simulink model "ClosedLoop"  (R2018b)
settings: Solver=VariableStepAuto  StartTime=0.0  StopTime=10  RelTol=1e-3
libraries: neural x533
(part 6 of 24)

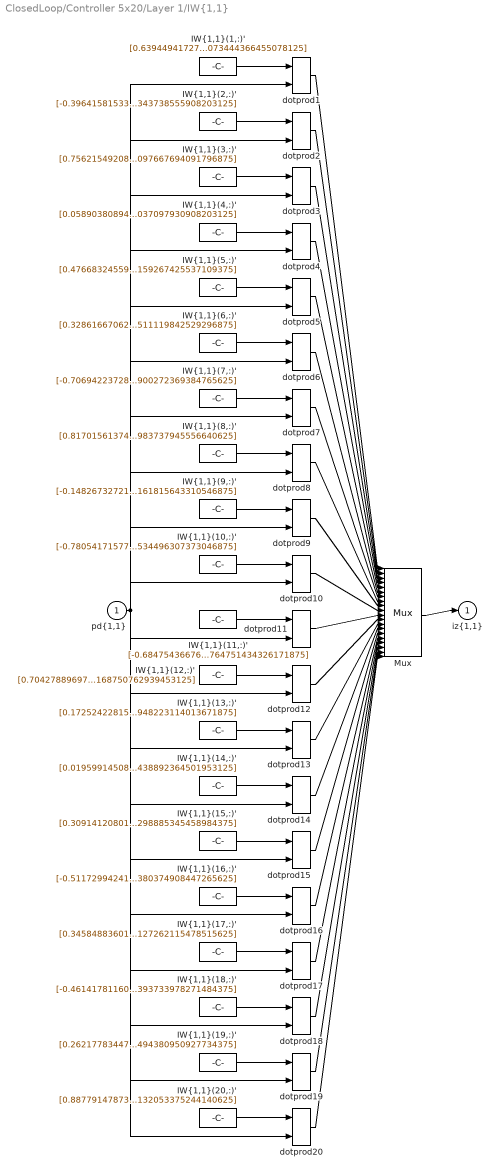
== system ClosedLoop/Controller 5x20/Layer 1/IW{1,1} ==
  "pd{1,1}" : Inport  PortDimensions=5
      mask Display: e = 0.06;c1 = [120 230 180]/255;c2 = ([120 230 180]+0)/(256+128);c3 = ([120 230 180]+128)/(256+128);patch([0 1 1 0],[0 0 1 1],c1);patch([0 1 1 1-e 1-e 0+e],[0 0 1 1-e 0+e 0+e],c2);patch([0 0 1 1-e 0+e 0+e],[0 1 1 1-e 1-e 0+e],c3);plot([0 1 1 0 0],[0 0 1 1 0]);
  "IW{1,1}(1,:)'" : Constant  Value=[0.63944941727794779584570505903684534132480621337890625;0.441873982701390388694306921024690382182598114013671875;0.1810593625517409321901141083799302577972412109375;-0.288327270168069638156538303519482724368572235107421875;-0.427441282480707507307471360036288388073444366455078125]
      mask Display: e = 0.06;c1 = [120 150 230]/255;c2 = ([120 150 230]+0)/383;c3 = ([120 150 230]+128)/383;patch([0 1 1 0],[0 0 1 1],c1);patch([0 1 1 1-e 1-e 0+e],[0 0 1 1-e 0+e 0+e],c2);patch([0 0 1 1-e 0+e 0+e],[0 1 1 1-e 1-e 0+e],c3);plot([0 1 1 0 0],[0 0 1 1 0]);disp('Weights');
  "IW{1,1}(10,:)'" : Constant  Value=[-0.780541715777256950303808480384759604930877685546875;0.64768264751365112186221040246891789138317108154296875;0.0832744460106624728723545558750629425048828125;0.52460666987157733576196960711968131363391876220703125;0.01510391606472875729305638259347688290290534496307373046875]
      mask Display: e = 0.06;c1 = [120 150 230]/255;c2 = ([120 150 230]+0)/383;c3 = ([120 150 230]+128)/383;patch([0 1 1 0],[0 0 1 1],c1);patch([0 1 1 1-e 1-e 0+e],[0 0 1 1-e 0+e 0+e],c2);patch([0 0 1 1-e 0+e 0+e],[0 1 1 1-e 1-e 0+e],c3);plot([0 1 1 0 0],[0 0 1 1 0]);disp('Weights');
  "IW{1,1}(11,:)'" : Constant  Value=[-0.68475436676158640825207157831755466759204864501953125;-0.357319180860754148643110283956048078835010528564453125;-0.6134220048648766354659755961620248854160308837890625;-0.55516072875852484624914495725533924996852874755859375;-0.47606734988326493418497875609318725764751434326171875]
      mask Display: e = 0.06;c1 = [120 150 230]/255;c2 = ([120 150 230]+0)/383;c3 = ([120 150 230]+128)/383;patch([0 1 1 0],[0 0 1 1],c1);patch([0 1 1 1-e 1-e 0+e],[0 0 1 1-e 0+e 0+e],c2);patch([0 0 1 1-e 0+e 0+e],[0 1 1 1-e 1-e 0+e],c3);plot([0 1 1 0 0],[0 0 1 1 0]);disp('Weights');
  "IW{1,1}(12,:)'" : Constant  Value=[0.70427889697472767505104229712742380797863006591796875;0.30288422449172036632347726481384597718715667724609375;-0.0523751521182032886425616879932931624352931976318359375;0.6147646637613533027177936673979274928569793701171875;0.41756010873698035101853065498289652168750762939453125]
      mask Display: e = 0.06;c1 = [120 150 230]/255;c2 = ([120 150 230]+0)/383;c3 = ([120 150 230]+128)/383;patch([0 1 1 0],[0 0 1 1],c1);patch([0 1 1 1-e 1-e 0+e],[0 0 1 1-e 0+e 0+e],c2);patch([0 0 1 1-e 0+e 0+e],[0 1 1 1-e 1-e 0+e],c3);plot([0 1 1 0 0],[0 0 1 1 0]);disp('Weights');
  "IW{1,1}(13,:)'" : Constant  Value=[0.172524228158408454714134450114215724170207977294921875;0.01229162079763308247637443315625205286778509616851806640625;-0.73979290215458792800973242265172302722930908203125;0.249500982539548832317422011328744702041149139404296875;-0.57950215730051979345915924568544141948223114013671875]
      mask Display: e = 0.06;c1 = [120 150 230]/255;c2 = ([120 150 230]+0)/383;c3 = ([120 150 230]+128)/383;patch([0 1 1 0],[0 0 1 1],c1);patch([0 1 1 1-e 1-e 0+e],[0 0 1 1-e 0+e 0+e],c2);patch([0 0 1 1-e 0+e 0+e],[0 1 1 1-e 1-e 0+e],c3);plot([0 1 1 0 0],[0 0 1 1 0]);disp('Weights');
  "IW{1,1}(14,:)'" : Constant  Value=[0.01959914508530875842939877884418820030987262725830078125;-0.682683523295935845709436762263067066669464111328125;-0.254846757327596928899282602287712506949901580810546875;-0.470498201017735373508088514427072368562221527099609375;-0.402036750942489196081197633247938938438892364501953125]
      mask Display: e = 0.06;c1 = [120 150 230]/255;c2 = ([120 150 230]+0)/383;c3 = ([120 150 230]+128)/383;patch([0 1 1 0],[0 0 1 1],c1);patch([0 1 1 1-e 1-e 0+e],[0 0 1 1-e 0+e 0+e],c2);patch([0 0 1 1-e 0+e 0+e],[0 1 1 1-e 1-e 0+e],c3);plot([0 1 1 0 0],[0 0 1 1 0]);disp('Weights');
  "IW{1,1}(15,:)'" : Constant  Value=[0.30914120801182909392679221127764321863651275634765625;-0.3889526490302082084582480092649348080158233642578125;-0.630260952151780795560398473753593862056732177734375;0.50292774374151016925083013120456598699092864990234375;0.60317210715845648305588611037819646298885345458984375]
      mask Display: e = 0.06;c1 = [120 150 230]/255;c2 = ([120 150 230]+0)/383;c3 = ([120 150 230]+128)/383;patch([0 1 1 0],[0 0 1 1],c1);patch([0 1 1 1-e 1-e 0+e],[0 0 1 1-e 0+e 0+e],c2);patch([0 0 1 1-e 0+e 0+e],[0 1 1 1-e 1-e 0+e],c3);plot([0 1 1 0 0],[0 0 1 1 0]);disp('Weights');
  "IW{1,1}(16,:)'" : Constant  Value=[-0.511729942413364558007060622912831604480743408203125;-0.787376548696963052265118676587007939815521240234375;-0.11594008500043440079707579570822417736053466796875;0.5099989427324824742271403010818175971508026123046875;-0.8678719459485453313618563697673380374908447265625]
      mask Display: e = 0.06;c1 = [120 150 230]/255;c2 = ([120 150 230]+0)/383;c3 = ([120 150 230]+128)/383;patch([0 1 1 0],[0 0 1 1],c1);patch([0 1 1 1-e 1-e 0+e],[0 0 1 1-e 0+e 0+e],c2);patch([0 0 1 1-e 0+e 0+e],[0 1 1 1-e 1-e 0+e],c3);plot([0 1 1 0 0],[0 0 1 1 0]);disp('Weights');
  "IW{1,1}(17,:)'" : Constant  Value=[0.345848836012182137000792181424912996590137481689453125;0.739192252870459309832540384377352893352508544921875;0.3498306369600612253378812965820543467998504638671875;-0.67389569935591275839925629043136723339557647705078125;-0.81931527679271454189802170731127262115478515625]
      mask Display: e = 0.06;c1 = [120 150 230]/255;c2 = ([120 150 230]+0)/383;c3 = ([120 150 230]+128)/383;patch([0 1 1 0],[0 0 1 1],c1);patch([0 1 1 1-e 1-e 0+e],[0 0 1 1-e 0+e 0+e],c2);patch([0 0 1 1-e 0+e 0+e],[0 1 1 1-e 1-e 0+e],c3);plot([0 1 1 0 0],[0 0 1 1 0]);disp('Weights');
  "IW{1,1}(18,:)'" : Constant  Value=[-0.461417811606915362343528386190882883965969085693359375;0.36009780194955587351302028764621354639530181884765625;0.455915914545793665713091513680410571396350860595703125;-0.544014077344936897162597233545966446399688720703125;-0.12183088722031230888287467450936674140393733978271484375]
      mask Display: e = 0.06;c1 = [120 150 230]/255;c2 = ([120 150 230]+0)/383;c3 = ([120 150 230]+128)/383;patch([0 1 1 0],[0 0 1 1],c1);patch([0 1 1 1-e 1-e 0+e],[0 0 1 1-e 0+e 0+e],c2);patch([0 0 1 1-e 0+e 0+e],[0 1 1 1-e 1-e 0+e],c3);plot([0 1 1 0 0],[0 0 1 1 0]);disp('Weights');
  "IW{1,1}(19,:)'" : Constant  Value=[0.262177834471462090082383156186551786959171295166015625;0.6535154375374367941020636862958781421184539794921875;0.6456369613768373483253526501357555389404296875;0.1968913395570332791617573775511118583381175994873046875;-0.6650617297993670629097096025361679494380950927734375]
      mask Display: e = 0.06;c1 = [120 150 230]/255;c2 = ([120 150 230]+0)/383;c3 = ([120 150 230]+128)/383;patch([0 1 1 0],[0 0 1 1],c1);patch([0 1 1 1-e 1-e 0+e],[0 0 1 1-e 0+e 0+e],c2);patch([0 0 1 1-e 0+e 0+e],[0 1 1 1-e 1-e 0+e],c3);plot([0 1 1 0 0],[0 0 1 1 0]);disp('Weights');
  "IW{1,1}(2,:)'" : Constant  Value=[-0.39641581533467740161569281553965993225574493408203125;0.94362771281294233194358866967377252876758575439453125;-0.0251969357247785845366205847994933719746768474578857421875;0.63069245720279820677234283721190877258777618408203125;0.46812222722309126954343128090840764343738555908203125]
      mask Display: e = 0.06;c1 = [120 150 230]/255;c2 = ([120 150 230]+0)/383;c3 = ([120 150 230]+128)/383;patch([0 1 1 0],[0 0 1 1],c1);patch([0 1 1 1-e 1-e 0+e],[0 0 1 1-e 0+e 0+e],c2);patch([0 0 1 1-e 0+e 0+e],[0 1 1 1-e 1-e 0+e],c3);plot([0 1 1 0 0],[0 0 1 1 0]);disp('Weights');
  "IW{1,1}(20,:)'" : Constant  Value=[0.88779147873542996194373699836432933807373046875;0.89062236195547728190291536520817317068576812744140625;0.49647128185477729100938404371845535933971405029296875;-0.36536568262290092246047379376250319182872772216796875;0.92081085437169252205791281085112132132053375244140625]
      mask Display: e = 0.06;c1 = [120 150 230]/255;c2 = ([120 150 230]+0)/383;c3 = ([120 150 230]+128)/383;patch([0 1 1 0],[0 0 1 1],c1);patch([0 1 1 1-e 1-e 0+e],[0 0 1 1-e 0+e 0+e],c2);patch([0 0 1 1-e 0+e 0+e],[0 1 1 1-e 1-e 0+e],c3);plot([0 1 1 0 0],[0 0 1 1 0]);disp('Weights');
  "IW{1,1}(3,:)'" : Constant  Value=[0.75621549208736305036637759258155710995197296142578125;0.52112681140457706163715556613169610500335693359375;0.15712176310640912912930389211396686732769012451171875;0.03477553145685263746855753197451122105121612548828125;0.152933664299456484325645533317583613097667694091796875]
      mask Display: e = 0.06;c1 = [120 150 230]/255;c2 = ([120 150 230]+0)/383;c3 = ([120 150 230]+128)/383;patch([0 1 1 0],[0 0 1 1],c1);patch([0 1 1 1-e 1-e 0+e],[0 0 1 1-e 0+e 0+e],c2);patch([0 0 1 1-e 0+e 0+e],[0 1 1 1-e 1-e 0+e],c3);plot([0 1 1 0 0],[0 0 1 1 0]);disp('Weights');
  "IW{1,1}(4,:)'" : Constant  Value=[0.05890380894817469348279104224275215528905391693115234375;0.047611677570757814093038717828676453791558742523193359375;0.7530116683399459276415655040182173252105712890625;-0.331442609125007392467665567892254330217838287353515625;0.2493135330344113942402373140794225037097930908203125]
      mask Display: e = 0.06;c1 = [120 150 230]/255;c2 = ([120 150 230]+0)/383;c3 = ([120 150 230]+128)/383;patch([0 1 1 0],[0 0 1 1],c1);patch([0 1 1 1-e 1-e 0+e],[0 0 1 1-e 0+e 0+e],c2);patch([0 0 1 1-e 0+e 0+e],[0 1 1 1-e 1-e 0+e],c3);plot([0 1 1 0 0],[0 0 1 1 0]);disp('Weights');
  "IW{1,1}(5,:)'" : Constant  Value=[0.476683245594003490719359206195804290473461151123046875;-0.106451544391355901186813071035430766642093658447265625;0.1983172569855511102598910611050087027251720428466796875;-0.5240244069983972519111148358206264674663543701171875;0.301396811275104814509262496358132921159267425537109375]
      mask Display: e = 0.06;c1 = [120 150 230]/255;c2 = ([120 150 230]+0)/383;c3 = ([120 150 230]+128)/383;patch([0 1 1 0],[0 0 1 1],c1);patch([0 1 1 1-e 1-e 0+e],[0 0 1 1-e 0+e 0+e],c2);patch([0 0 1 1-e 0+e 0+e],[0 1 1 1-e 1-e 0+e],c3);plot([0 1 1 0 0],[0 0 1 1 0]);disp('Weights');
  "IW{1,1}(6,:)'" : Constant  Value=[0.32861667062527966098883780432515777647495269775390625;0.27485617132566220188749639419256709516048431396484375;0.670903154829147752025164663791656494140625;-0.8379688517272267933577722942573018372058868408203125;0.8012625535086701500375738760340027511119842529296875]
      mask Display: e = 0.06;c1 = [120 150 230]/255;c2 = ([120 150 230]+0)/383;c3 = ([120 150 230]+128)/383;patch([0 1 1 0],[0 0 1 1],c1);patch([0 1 1 1-e 1-e 0+e],[0 0 1 1-e 0+e 0+e],c2);patch([0 0 1 1-e 0+e 0+e],[0 1 1 1-e 1-e 0+e],c3);plot([0 1 1 0 0],[0 0 1 1 0]);disp('Weights');
  "IW{1,1}(7,:)'" : Constant  Value=[-0.70694223728522109784222493544803000986576080322265625;-0.38508756869127480637615690284292213618755340576171875;-0.0229183744784411912165378311101449071429669857025146484375;-0.57443912376093375637964300040039233863353729248046875;-0.59805450015968253385523212273255921900272369384765625]
      mask Display: e = 0.06;c1 = [120 150 230]/255;c2 = ([120 150 230]+0)/383;c3 = ([120 150 230]+128)/383;patch([0 1 1 0],[0 0 1 1],c1);patch([0 1 1 1-e 1-e 0+e],[0 0 1 1-e 0+e 0+e],c2);patch([0 0 1 1-e 0+e 0+e],[0 1 1 1-e 1-e 0+e],c3);plot([0 1 1 0 0],[0 0 1 1 0]);disp('Weights');
  "IW{1,1}(8,:)'" : Constant  Value=[0.81701561374423203876204979678732343018054962158203125;-0.11925247272886185800899738751468248665332794189453125;-0.8148800409285461565644936854369007050991058349609375;0.6699379370098370589658998142112977802753448486328125;0.2413222105500209269113298660158761776983737945556640625]
      mask Display: e = 0.06;c1 = [120 150 230]/255;c2 = ([120 150 230]+0)/383;c3 = ([120 150 230]+128)/383;patch([0 1 1 0],[0 0 1 1],c1);patch([0 1 1 1-e 1-e 0+e],[0 0 1 1-e 0+e 0+e],c2);patch([0 0 1 1-e 0+e 0+e],[0 1 1 1-e 1-e 0+e],c3);plot([0 1 1 0 0],[0 0 1 1 0]);disp('Weights');
  "IW{1,1}(9,:)'" : Constant  Value=[-0.1482673272100884231949891045587719418108463287353515625;0.33066414110135788906319476154749281704425811767578125;-0.423695552459811330958672215274418704211711883544921875;-0.62673649043667634117582565522752702236175537109375;-0.04549208932538333083339665563471498899161815643310546875]
      mask Display: e = 0.06;c1 = [120 150 230]/255;c2 = ([120 150 230]+0)/383;c3 = ([120 150 230]+128)/383;patch([0 1 1 0],[0 0 1 1],c1);patch([0 1 1 1-e 1-e 0+e],[0 0 1 1-e 0+e 0+e],c2);patch([0 0 1 1-e 0+e 0+e],[0 1 1 1-e 1-e 0+e],c3);plot([0 1 1 0 0],[0 0 1 1 0]);disp('Weights');
  Mux : Mux  Inputs=20
      mask Display: e = 0.06;c1 = [120 150 230]/255;c2 = ([120 150 230]+0)/383;c3 = ([120 150 230]+128)/383;patch([0 1 1 0],[0 0 1 1],c1);patch([0 1 1 1-e 1-e 0+e],[0 0 1 1-e 0+e 0+e],c2);patch([0 0 1 1-e 0+e 0+e],[0 1 1 1-e 1-e 0+e],c3);plot([0 1 1 0 0],[0 0 1 1 0]);disp('Mux');
  dotprod{1..20} (20 alike) : neural/Weight Functions/dotprod
  "iz{1,1}" : Outport
      mask Display: e = 0.06;c1 = [120 230 180]/255;c2 = ([120 230 180]+0)/(256+128);c3 = ([120 230 180]+128)/(256+128);patch([0 1 1 0],[0 0 1 1],c1);patch([0 1 1 1-e 1-e 0+e],[0 0 1 1-e 0+e 0+e],c2);patch([0 0 1 1-e 0+e 0+e],[0 1 1 1-e 1-e 0+e],c3);plot([0 1 1 0 0],[0 0 1 1 0]);
  wires:
  Mux/1 -> "iz{1,1}"/1
  dotprod20/1 -> Mux/20
  "IW{1,1}(20,:)'"/1 -> dotprod20/1
  dotprod19/1 -> Mux/19
  "IW{1,1}(19,:)'"/1 -> dotprod19/1
  dotprod18/1 -> Mux/18
  "IW{1,1}(18,:)'"/1 -> dotprod18/1
  dotprod17/1 -> Mux/17
  "IW{1,1}(17,:)'"/1 -> dotprod17/1
  dotprod16/1 -> Mux/16
  "IW{1,1}(16,:)'"/1 -> dotprod16/1
  dotprod15/1 -> Mux/15
  "IW{1,1}(15,:)'"/1 -> dotprod15/1
  dotprod14/1 -> Mux/14
  "IW{1,1}(14,:)'"/1 -> dotprod14/1
  dotprod13/1 -> Mux/13
  "IW{1,1}(13,:)'"/1 -> dotprod13/1
  dotprod12/1 -> Mux/12
  "IW{1,1}(12,:)'"/1 -> dotprod12/1
  dotprod11/1 -> Mux/11
  "IW{1,1}(11,:)'"/1 -> dotprod11/1
  dotprod10/1 -> Mux/10
  "IW{1,1}(10,:)'"/1 -> dotprod10/1
  dotprod9/1 -> Mux/9
  "IW{1,1}(9,:)'"/1 -> dotprod9/1
  dotprod8/1 -> Mux/8
  "IW{1,1}(8,:)'"/1 -> dotprod8/1
  dotprod7/1 -> Mux/7
  "IW{1,1}(7,:)'"/1 -> dotprod7/1
  dotprod6/1 -> Mux/6
  "IW{1,1}(6,:)'"/1 -> dotprod6/1
  dotprod5/1 -> Mux/5
  "IW{1,1}(5,:)'"/1 -> dotprod5/1
  dotprod4/1 -> Mux/4
  "IW{1,1}(4,:)'"/1 -> dotprod4/1
  dotprod3/1 -> Mux/3
  "IW{1,1}(3,:)'"/1 -> dotprod3/1
  dotprod2/1 -> Mux/2
  "IW{1,1}(2,:)'"/1 -> dotprod2/1
  dotprod1/1 -> Mux/1
  "pd{1,1}"/1 -> dotprod20/2, dotprod19/2, dotprod18/2, dotprod17/2, dotprod16/2, dotprod15/2, dotprod14/2, dotprod13/2, dotprod12/2, dotprod11/2, dotprod10/2, dotprod9/2, dotprod8/2, dotprod7/2, dotprod6/2, dotprod5/2, dotprod4/2, dotprod3/2, dotprod2/2, dotprod1/2
  "IW{1,1}(1,:)'"/1 -> dotprod1/1

== system ClosedLoop/Controller 5x20/Layer 2/Delays 1 ==
  "p{2}" : Inport  PortDimensions=20
      mask Display: e = 0.06;c1 = [120 230 180]/255;c2 = ([120 230 180]+0)/(256+128);c3 = ([120 230 180]+128)/(256+128);patch([0 1 1 0],[0 0 1 1],c1);patch([0 1 1 1-e 1-e 0+e],[0 0 1 1-e 0+e 0+e],c2);patch([0 0 1 1-e 0+e 0+e],[0 1 1 1-e 1-e 0+e],c3);plot([0 1 1 0 0],[0 0 1 1 0]);
  mux : Mux  Inputs=1
      mask Display: e = 0.06;c1 = [120 150 230]/255;c2 = ([120 150 230]+0)/383;c3 = ([120 150 230]+128)/383;patch([0 1 1 0],[0 0 1 1],c1);patch([0 1 1 1-e 1-e 0+e],[0 0 1 1-e 0+e 0+e],c2);patch([0 0 1 1-e 0+e 0+e],[0 1 1 1-e 1-e 0+e],c3);plot([0 1 1 0 0],[0 0 1 1 0]);disp('Mux')
  "pd{2,1}" : Outport
      mask Display: e = 0.06;c1 = [120 230 180]/255;c2 = ([120 230 180]+0)/(256+128);c3 = ([120 230 180]+128)/(256+128);patch([0 1 1 0],[0 0 1 1],c1);patch([0 1 1 1-e 1-e 0+e],[0 0 1 1-e 0+e 0+e],c2);patch([0 0 1 1-e 0+e 0+e],[0 1 1 1-e 1-e 0+e],c3);plot([0 1 1 0 0],[0 0 1 1 0]);
  wires:
  mux/1 -> "pd{2,1}"/1
  "p{2}"/1 -> mux/1

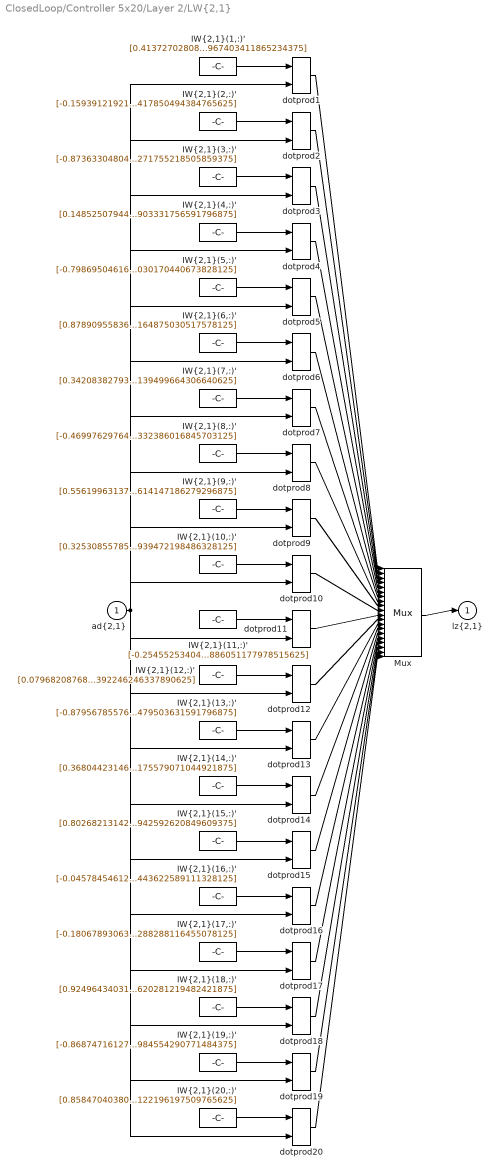
== system ClosedLoop/Controller 5x20/Layer 2/LW{2,1} ==
  "ad{2,1}" : Inport  PortDimensions=20
      mask Display: e = 0.06;c1 = [120 230 180]/255;c2 = ([120 230 180]+0)/(256+128);c3 = ([120 230 180]+128)/(256+128);patch([0 1 1 0],[0 0 1 1],c1);patch([0 1 1 1-e 1-e 0+e],[0 0 1 1-e 0+e 0+e],c2);patch([0 0 1 1-e 0+e 0+e],[0 1 1 1-e 1-e 0+e],c3);plot([0 1 1 0 0],[0 0 1 1 0]);
  "IW{2,1}(1,:)'" : Constant  Value=[0.41372702808061634360825564726837910711765289306640625;0.62068992936244882230312214232981204986572265625;-0.3914076908031651758079760838882066309452056884765625;-0.1273624055136741428650992702387156896293163299560546875;0.4630783512187885975208700983785092830657958984375;0.5398937278440520959321702321176417171955108642578125;-0.50464881122157134729633298775297589600086212158203125;0.54020295173985932724036729268846102058887481689453125;0.1306628996043121826442501287601771764457225799560546875;-0.52058594370764954550878655936685390770435333251953125;0.2408992494088320335254849169359658844769001007080078125;0.6600151299617120770335532142780721187591552734375;0.931678784682436589292819917318411171436309814453125;0.1519514250811669076046683812819537706673145294189453125;0.0864028325093663396305743162884027697145938873291015625;-0.30186150825793145457964783417992293834686279296875;0.1461560366215612638551846202972228638827800750732421875;0.6573024051289804159381446879706345498561859130859375;-0.344777445692799056065069862597738392651081085205078125;-0.23891590200468593163662944789393804967403411865234375]
      mask Display: e = 0.06;c1 = [120 150 230]/255;c2 = ([120 150 230]+0)/383;c3 = ([120 150 230]+128)/383;patch([0 1 1 0],[0 0 1 1],c1);patch([0 1 1 1-e 1-e 0+e],[0 0 1 1-e 0+e 0+e],c2);patch([0 0 1 1-e 0+e 0+e],[0 1 1 1-e 1-e 0+e],c3);plot([0 1 1 0 0],[0 0 1 1 0]);disp('weights');
  "IW{2,1}(10,:)'" : Constant  Value=[0.3253085578530334753821762205916456878185272216796875;-0.304829756998219403296701557337655685842037200927734375;0.88010133984902816361994837279780767858028411865234375;0.8416425234628761575805810934980399906635284423828125;0.56110125378272523999356735657784156501293182373046875;-0.1701061698336301108991364117173361591994762420654296875;0.184820626777829677411801867492613382637500762939453125;-0.321484634075885067350242252359748817980289459228515625;-0.1468893135594261101228852339772856794297695159912109375;-0.83629443998785368830084507862920872867107391357421875;-0.17319307645534409711984835666953586041927337646484375;-0.2284721369925456768701366172535927034914493560791015625;-0.59150163914379938479015663688187487423419952392578125;-0.53715545432883404775026292554684914648532867431640625;-0.289680547942036792363751374068669974803924560546875;0.7642401916590857435807038200437091290950775146484375;0.63183866356985929346734565115184523165225982666015625;-0.255987405397600620293729889453970827162265777587890625;-0.69569101632231455933919050949043594300746917724609375;-0.2505679914805398755817122946609742939472198486328125]
      mask Display: e = 0.06;c1 = [120 150 230]/255;c2 = ([120 150 230]+0)/383;c3 = ([120 150 230]+128)/383;patch([0 1 1 0],[0 0 1 1],c1);patch([0 1 1 1-e 1-e 0+e],[0 0 1 1-e 0+e 0+e],c2);patch([0 0 1 1-e 0+e 0+e],[0 1 1 1-e 1-e 0+e],c3);plot([0 1 1 0 0],[0 0 1 1 0]);disp('weights');
  "IW{2,1}(11,:)'" : Constant  Value=[-0.254552534046267264766783000595751218497753143310546875;0.43378976888941622735984537939657457172870635986328125;-0.1176442810962321783296857802270096726715564727783203125;-1.0588629229904962247843513978295959532260894775390625;0.326115348711636332534880011735367588698863983154296875;0.4050434179513084931301136748516000807285308837890625;0.005118799549225894196524677681736648082733154296875;0.38040027546355725807103453917079605162143707275390625;-0.1722011339177583477688671109717688523232936859130859375;1.0572289522118343274570406720158644020557403564453125;-0.7943570490662386074376399847096763551235198974609375;0.339881641550732915835197900378261692821979522705078125;-0.467660054786290857453678881938685663044452667236328125;0.98889919394350889181311003994778729975223541259765625;0.0264857269062730264763683152295925538055598735809326171875;-0.362255471530811501423841036739759147167205810546875;0.12371218484571504248048512408786336891353130340576171875;-0.94436447378172427846720893285237252712249755859375;-0.062331148537743415183332018614237313158810138702392578125;-0.8106189575078401876595535213709808886051177978515625]
      mask Display: e = 0.06;c1 = [120 150 230]/255;c2 = ([120 150 230]+0)/383;c3 = ([120 150 230]+128)/383;patch([0 1 1 0],[0 0 1 1],c1);patch([0 1 1 1-e 1-e 0+e],[0 0 1 1-e 0+e 0+e],c2);patch([0 0 1 1-e 0+e 0+e],[0 1 1 1-e 1-e 0+e],c3);plot([0 1 1 0 0],[0 0 1 1 0]);disp('weights');
  "IW{2,1}(12,:)'" : Constant  Value=[0.07968208768754482529406146795736276544630527496337890625;0.041047636341366565415622602586154243908822536468505859375;0.416829252063110666792766778598888777196407318115234375;0.45312308547610502529323639464564621448516845703125;0.52333170533999517903822606967878527939319610595703125;0.71153805493735922116371739321039058268070220947265625;0.56576234985935280885627207680954597890377044677734375;-0.57822113492932125655698882837896235287189483642578125;-0.2211337561088375924800430993855115957558155059814453125;0.08542118951623108025206221327607636339962482452392578125;-0.400687559387449210301923585575423203408718109130859375;-0.50820358056139058877676006886758841574192047119140625;-0.1890455149757010733235773614069330506026744842529296875;0.413947184026870473871895228512585163116455078125;-0.9598825835539190887146787645178847014904022216796875;0.662459316041985601941632921807467937469482421875;-0.62227115521360565342234849595115520060062408447265625;0.12551069318583996103910749297938309609889984130859375;0.2428357344045399546228480858189868740737438201904296875;-0.434529047386081723747253136025392450392246246337890625]
      mask Display: e = 0.06;c1 = [120 150 230]/255;c2 = ([120 150 230]+0)/383;c3 = ([120 150 230]+128)/383;patch([0 1 1 0],[0 0 1 1],c1);patch([0 1 1 1-e 1-e 0+e],[0 0 1 1-e 0+e 0+e],c2);patch([0 0 1 1-e 0+e 0+e],[0 1 1 1-e 1-e 0+e],c3);plot([0 1 1 0 0],[0 0 1 1 0]);disp('weights');
  "IW{2,1}(13,:)'" : Constant  Value=[-0.8795678557672308439663311219192110002040863037109375;0.2437785652369919286996946539147756993770599365234375;0.0489167205949755656835264971959986723959445953369140625;-0.2029642793702139957900953959324397146701812744140625;0.2359428808879183436797433159881620667874813079833984375;0.329546789606764978231012719334103167057037353515625;0.420703845487026217853099296917207539081573486328125;0.86279288068060167038453300847322680056095123291015625;-0.445770225211319204294824203316238708794116973876953125;-0.51039401437666154226491244116914458572864532470703125;0.1045436501606975543410271711763925850391387939453125;-0.62926642345067573813821582007221877574920654296875;-1.016975422520903560297256262856535613536834716796875;-0.563819330421016839949288623756729066371917724609375;0.034476515022731142601220000187822734005749225616455078125;0.1803171532989119307810454984064563177525997161865234375;-0.7129578188773819658052843806217424571514129638671875;0.4626104593894038163881532454979605972766876220703125;-0.7199562722305146156287491976399905979633331298828125;-0.7456830468502442244016492622904479503631591796875]
      mask Display: e = 0.06;c1 = [120 150 230]/255;c2 = ([120 150 230]+0)/383;c3 = ([120 150 230]+128)/383;patch([0 1 1 0],[0 0 1 1],c1);patch([0 1 1 1-e 1-e 0+e],[0 0 1 1-e 0+e 0+e],c2);patch([0 0 1 1-e 0+e 0+e],[0 1 1 1-e 1-e 0+e],c3);plot([0 1 1 0 0],[0 0 1 1 0]);disp('weights');
  "IW{2,1}(14,:)'" : Constant  Value=[0.3680442314658873836918928645900450646877288818359375;0.5279084956297481756593015234102495014667510986328125;-0.412080206627506051564324707214836962521076202392578125;0.349719774151550755192374708713032305240631103515625;-0.3116898065406987772263391889282502233982086181640625;-0.157659777141759327445669214284862391650676727294921875;0.051592964153606708788135648546813172288239002227783203125;-0.9421416421161967758024502472835592925548553466796875;-0.59275925203621204762072238736436702311038970947265625;-0.71191078887096048699589800889953039586544036865234375;0.381375928788659612767020234969095326960086822509765625;-0.5503366868102246289851109395385719835758209228515625;-0.1003136642517905297022906552228960208594799041748046875;0.26451257211458301110695856550591997802257537841796875;0.92548485880867392694426598609425127506256103515625;0.06858222016657743169698591145788668654859066009521484375;0.538877078924025365580519064678810536861419677734375;0.2781545384253185648759654213790781795978546142578125;-0.020119346106335304902312799413266475312411785125732421875;0.622709933646842017651579226367175579071044921875]
      mask Display: e = 0.06;c1 = [120 150 230]/255;c2 = ([120 150 230]+0)/383;c3 = ([120 150 230]+128)/383;patch([0 1 1 0],[0 0 1 1],c1);patch([0 1 1 1-e 1-e 0+e],[0 0 1 1-e 0+e 0+e],c2);patch([0 0 1 1-e 0+e 0+e],[0 1 1 1-e 1-e 0+e],c3);plot([0 1 1 0 0],[0 0 1 1 0]);disp('weights');
  "IW{2,1}(15,:)'" : Constant  Value=[0.80268213142427857764715781740960665047168731689453125;-0.58198971361380547051567191374488174915313720703125;-0.9886476994639463722336358841857872903347015380859375;-0.84541346302483855179588090322795324027538299560546875;-0.675026282750535333576635821373201906681060791015625;0.582061519441452901446609757840633392333984375;-0.69713975855702103867628238731413148343563079833984375;-0.054850803783529973600696649782548774965107440948486328125;0.471421280151244903589002888111281208693981170654296875;-0.86839672369021869702265803425689227879047393798828125;-0.33059801164834345943432936110184527933597564697265625;-0.383310836448245539909152057589381001889705657958984375;-1.02188824896290242350005428306758403778076171875;-0.72448580936499362703528959173127077519893646240234375;-0.06797784462999569010666078838767134584486484527587890625;0.67420876504152171815320571113261394202709197998046875;0.2468461351802111736208900083511252887547016143798828125;-0.84093529499425356821262766970903612673282623291015625;0.53307619750418944182257519059930928051471710205078125;0.188779459207717825730554750407463870942592620849609375]
      mask Display: e = 0.06;c1 = [120 150 230]/255;c2 = ([120 150 230]+0)/383;c3 = ([120 150 230]+128)/383;patch([0 1 1 0],[0 0 1 1],c1);patch([0 1 1 1-e 1-e 0+e],[0 0 1 1-e 0+e 0+e],c2);patch([0 0 1 1-e 0+e 0+e],[0 1 1 1-e 1-e 0+e],c3);plot([0 1 1 0 0],[0 0 1 1 0]);disp('weights');
  "IW{2,1}(16,:)'" : Constant  Value=[-0.045784546129320848051325043570614070631563663482666015625;-0.01107750770821676333799388203260605223476886749267578125;-0.42067431995422499557690798610565252602100372314453125;0.552076430003165086191074806265532970428466796875;0.77175652837282593399237384801381267607212066650390625;-0.34650140055324618604259967469261027872562408447265625;0.1924341010435884624651947660822770558297634124755859375;0.265799404293726837522626738063991069793701171875;0.71978414257599221404149147929274477064609527587890625;-0.9484359638995953911688729931483976542949676513671875;0.059928585817393985324397220892933546565473079681396484375;-0.81073738131111727778232989294338040053844451904296875;-0.91058591264126154118940803527948446571826934814453125;0.072726710083328260925128461167332716286182403564453125;-0.297519645927611264824008685536682605743408203125;0.5759417392995882511996796893072314560413360595703125;-0.336522514322294907795907192848972044885158538818359375;-0.6284661325713376545110122606274671852588653564453125;-0.67773130163473371823101842892356216907501220703125;0.33137617823979070852402628588606603443622589111328125]
      mask Display: e = 0.06;c1 = [120 150 230]/255;c2 = ([120 150 230]+0)/383;c3 = ([120 150 230]+128)/383;patch([0 1 1 0],[0 0 1 1],c1);patch([0 1 1 1-e 1-e 0+e],[0 0 1 1-e 0+e 0+e],c2);patch([0 0 1 1-e 0+e 0+e],[0 1 1 1-e 1-e 0+e],c3);plot([0 1 1 0 0],[0 0 1 1 0]);disp('weights');
  "IW{2,1}(17,:)'" : Constant  Value=[-0.1806789306391623217695752146028098650276660919189453125;0.45123067495923530056955996769829653203487396240234375;0.3288746629019823064510319454711861908435821533203125;-0.74350581279448046956304096966050565242767333984375;0.76508328881713938418585030376561917364597320556640625;-0.55823380357217400327130008008680306375026702880859375;0.83037082608507273295828099435311742126941680908203125;-0.039984093042162605069478331643040291965007781982421875;0.583199456912266267494260318926535546779632568359375;-0.316009428932014502233727171187638305127620697021484375;0.2330453160915997024016377281441236846148967742919921875;0.1858422832673997382446628989782766439020633697509765625;-0.7414385229760209750082822210970334708690643310546875;0.513571609579043464322012368938885629177093505859375;0.457194499361955053462480691450764425098896026611328125;0.1462665782613894183139535698501276783645153045654296875;-0.71754133926725727210538252620608545839786529541015625;0.5720192236405685637379292529658414423465728759765625;0.251299625967165318751739278013701550662517547607421875;0.28301408073860034875224300776608288288116455078125]
      mask Display: e = 0.06;c1 = [120 150 230]/255;c2 = ([120 150 230]+0)/383;c3 = ([120 150 230]+128)/383;patch([0 1 1 0],[0 0 1 1],c1);patch([0 1 1 1-e 1-e 0+e],[0 0 1 1-e 0+e 0+e],c2);patch([0 0 1 1-e 0+e 0+e],[0 1 1 1-e 1-e 0+e],c3);plot([0 1 1 0 0],[0 0 1 1 0]);disp('weights');
  "IW{2,1}(18,:)'" : Constant  Value=[0.92496434031542784648394217583700083196163177490234375;-0.3612498407903836916688078417791984975337982177734375;-0.606433636955590049666398044792003929615020751953125;0.2148675706104379024008466103623504750430583953857421875;0.57330236524422117927457520636380650103092193603515625;-0.66588820872680332119131207946338690817356109619140625;0.832285547338539544170998851768672466278076171875;-0.74595763106272239273408786175423301756381988525390625;-0.807570969268340821400897766579873859882354736328125;0.1584556405316577265551813979982398450374603271484375;0.4849190697094358792895718579529784619808197021484375;0.8834810949073508279383304397924803197383880615234375;-0.521885351243142725508050716598518192768096923828125;-0.159138379881506419888381742566707544028759002685546875;-0.67138061761340439570489024845301173627376556396484375;-0.97205789202822912020707235569716431200504302978515625;-0.2301880659565917752740205060035805217921733856201171875;0.054335041171990026975802123843095614574849605560302734375;0.6482964478818169506979529614909552037715911865234375;0.0542879998960570098187616849827463738620281219482421875]
      mask Display: e = 0.06;c1 = [120 150 230]/255;c2 = ([120 150 230]+0)/383;c3 = ([120 150 230]+128)/383;patch([0 1 1 0],[0 0 1 1],c1);patch([0 1 1 1-e 1-e 0+e],[0 0 1 1-e 0+e 0+e],c2);patch([0 0 1 1-e 0+e 0+e],[0 1 1 1-e 1-e 0+e],c3);plot([0 1 1 0 0],[0 0 1 1 0]);disp('weights');
  "IW{2,1}(19,:)'" : Constant  Value=[-0.86874716127473583515694599554990418255329132080078125;0.5276507027260939342028223109082318842411041259765625;-0.5432759007095440129120333949686028063297271728515625;0.1378431129323197390501576364840730093419551849365234375;-0.263030959077549086888581086896010674536228179931640625;0.407323651402714592695275541700539179146289825439453125;0.446347152406902036858582505374215543270111083984375;0.3762307957115400558478768289205618202686309814453125;0.10863265857891679644353644107468426227569580078125;0.56448626612201469043839097139425575733184814453125;0.3877746604814957809281850131810642778873443603515625;0.528011658095508540355922377784736454486846923828125;0.213888240924233363760009751786128617823123931884765625;-0.8326711878777957043240576240350492298603057861328125;-0.78205950971029292162484125583432614803314208984375;-0.2435248748779113292517450872765039093792438507080078125;-0.0153651787458631179650314635409813490696251392364501953125;-0.2312618416720850778034446193487383425235748291015625;0.00184857992248182848894766383551768740289844572544097900390625;-0.53761299172847287763943313620984554290771484375]
      mask Display: e = 0.06;c1 = [120 150 230]/255;c2 = ([120 150 230]+0)/383;c3 = ([120 150 230]+128)/383;patch([0 1 1 0],[0 0 1 1],c1);patch([0 1 1 1-e 1-e 0+e],[0 0 1 1-e 0+e 0+e],c2);patch([0 0 1 1-e 0+e 0+e],[0 1 1 1-e 1-e 0+e],c3);plot([0 1 1 0 0],[0 0 1 1 0]);disp('weights');
  "IW{2,1}(2,:)'" : Constant  Value=[-0.1593912192117015458325823829000000841915607452392578125;0.6188142687233593175477608383516781032085418701171875;-0.00461547188775751800193791751780736376531422138214111328125;0.2995726849903015409637418997590430080890655517578125;-0.475313757213221055319962715657311491668224334716796875;-0.455706527800538940820018751765019260346889495849609375;0.92325014706478747417150998444412834942340850830078125;-0.7170428051471671171412936018896289169788360595703125;-0.197746479201530045433088389472686685621738433837890625;-0.140388591920281857738928010803647339344024658203125;-0.554679992596371018720446954830549657344818115234375;-0.261020094003090452616788752493448555469512939453125;-0.80549613572569278563406669491087086498737335205078125;0.08793817764785073765043676985442289151251316070556640625;-0.737250586887996828266977900057099759578704833984375;0.587324551962286278694591601379215717315673828125;-0.683062525553314703330443080631084740161895751953125;0.93397326024384452747284512952319346368312835693359375;0.9175565338587474695231094301561824977397918701171875;0.98080011750530238234802027363912202417850494384765625]
      mask Display: e = 0.06;c1 = [120 150 230]/255;c2 = ([120 150 230]+0)/383;c3 = ([120 150 230]+128)/383;patch([0 1 1 0],[0 0 1 1],c1);patch([0 1 1 1-e 1-e 0+e],[0 0 1 1-e 0+e 0+e],c2);patch([0 0 1 1-e 0+e 0+e],[0 1 1 1-e 1-e 0+e],c3);plot([0 1 1 0 0],[0 0 1 1 0]);disp('weights');
  "IW{2,1}(20,:)'" : Constant  Value=[0.858470403801856907222145309788174927234649658203125;0.3596152347934236104265437461435794830322265625;0.7552440559429693944792916227015666663646697998046875;0.0601795499082851126360083071631379425525665283203125;-0.00755023756927375444547578808851540088653564453125;-0.9490160527383924016220362318563275039196014404296875;-0.6248831317380967309560446665273047983646392822265625;-0.570837548710489084413666205364279448986053466796875;0.176348981656517356242375171859748661518096923828125;0.25350844363951186011263416730798780918121337890625;-0.7262389314713104671028531811316497623920440673828125;-0.517135555343453123811059413128532469272613525390625;-0.536555084148062189086658690939657390117645263671875;0.1742134412923512787330082574044354259967803955078125;-0.1091841483734883322398445670842193067073822021484375;-0.127758394510482542472118439036421477794647216796875;0.0710052871003028496232900579343549907207489013671875;-0.4233643555650024037362300077802501618862152099609375;-0.990372379820247061843474511988461017608642578125;-0.8053736847920609509543510284856893122196197509765625]
      mask Display: e = 0.06;c1 = [120 150 230]/255;c2 = ([120 150 230]+0)/383;c3 = ([120 150 230]+128)/383;patch([0 1 1 0],[0 0 1 1],c1);patch([0 1 1 1-e 1-e 0+e],[0 0 1 1-e 0+e 0+e],c2);patch([0 0 1 1-e 0+e 0+e],[0 1 1 1-e 1-e 0+e],c3);plot([0 1 1 0 0],[0 0 1 1 0]);disp('weights');
  "IW{2,1}(3,:)'" : Constant  Value=[-0.87363304804092367650270034573622979223728179931640625;0.6015407854511416463338946414296515285968780517578125;0.71376296530793081895893692490062676370143890380859375;-0.70090675964932380725969096602057106792926788330078125;-0.567101089765580379520315545960329473018646240234375;-0.5713248906354266853924173119594343006610870361328125;0.8860428882356912172468810240388847887516021728515625;0.56575657959649572337212930506211705505847930908203125;0.63466341541288073813120718114078044891357421875;0.523264647719439590645151838543824851512908935546875;-0.492624839572022354960978418603190220892429351806640625;0.09008088012467130312188601237721741199493408203125;0.54996767762660236922300782680395059287548065185546875;-0.327250171390309374519489438171149231493473052978515625;0.733626015813464871229143682285211980342864990234375;0.374162494434288672717769941300502978265285491943359375;0.09860924427790047908093384876337950117886066436767578125;-0.235189082410515393206651424407027661800384521484375;-0.206718935849254881187420096466667018830776214599609375;-0.73886986320788350379729081396362744271755218505859375]
      mask Display: e = 0.06;c1 = [120 150 230]/255;c2 = ([120 150 230]+0)/383;c3 = ([120 150 230]+128)/383;patch([0 1 1 0],[0 0 1 1],c1);patch([0 1 1 1-e 1-e 0+e],[0 0 1 1-e 0+e 0+e],c2);patch([0 0 1 1-e 0+e 0+e],[0 1 1 1-e 1-e 0+e],c3);plot([0 1 1 0 0],[0 0 1 1 0]);disp('weights');
  "IW{2,1}(4,:)'" : Constant  Value=[0.1485250794462278367547014568117447197437286376953125;-0.78336871745494451868552232554065994918346405029296875;-0.50268266389585658515670729684643447399139404296875;-0.4768186813436574578162208126741461455821990966796875;0.4997195087893124831879276825929991900920867919921875;-0.389101188545940057661454147819313220679759979248046875;1.015927427643496638864917258615605533123016357421875;-0.7622625353906469225506725706509314477443695068359375;0.77005288775988633975799757536151446402072906494140625;-0.3963287937092061508081997089902870357036590576171875;0.2116119957228065062704303045393317006528377532958984375;0.92529438728370283495650028271484188735485076904296875;-0.2911610634460493063357944265590049326419830322265625;0.998814952981231130024752928875386714935302734375;-0.07178905673158779421338948623088072054088115692138671875;0.06618065392293459581196657381951808929443359375;-0.22351428101298365103133392040035687386989593505859375;-0.62292311974734726476299329078756272792816162109375;-0.6423929217994130969060506686219014227390289306640625;0.53717328544357190178715200090664438903331756591796875]
      mask Display: e = 0.06;c1 = [120 150 230]/255;c2 = ([120 150 230]+0)/383;c3 = ([120 150 230]+128)/383;patch([0 1 1 0],[0 0 1 1],c1);patch([0 1 1 1-e 1-e 0+e],[0 0 1 1-e 0+e 0+e],c2);patch([0 0 1 1-e 0+e 0+e],[0 1 1 1-e 1-e 0+e],c3);plot([0 1 1 0 0],[0 0 1 1 0]);disp('weights');
  "IW{2,1}(5,:)'" : Constant  Value=[-0.7986950461681006085967737817554734647274017333984375;0.4538485799631255535047102966927923262119293212890625;-0.927626968286265896068698566523380577564239501953125;0.50415318774774797727644681799574755132198333740234375;0.81450682250085615354606716209673322737216949462890625;-0.261766557489906126487966275817598216235637664794921875;-0.866072068552302010147059263545088469982147216796875;0.1923910217514941123351235319205443374812602996826171875;0.560246184857401186008019067230634391307830810546875;-0.036308321049691789916824546935458783991634845733642578125;-0.33999526201654906021332180898752994835376739501953125;0.90367754620000184662131914592464454472064971923828125;-0.440036504827832020136924029429792426526546478271484375;-0.70791906433385032304528294844203628599643707275390625;-0.42434685570408081645155107253231108188629150390625;-0.57683208960559395617195832528523169457912445068359375;-0.83222961672620410222833697844180278480052947998046875;0.97439500746408935771825099436682648956775665283203125;0.022050937483775921721385060436659841798245906829833984375;-0.2402320011554579526347197315772064030170440673828125]
      mask Display: e = 0.06;c1 = [120 150 230]/255;c2 = ([120 150 230]+0)/383;c3 = ([120 150 230]+128)/383;patch([0 1 1 0],[0 0 1 1],c1);patch([0 1 1 1-e 1-e 0+e],[0 0 1 1-e 0+e 0+e],c2);patch([0 0 1 1-e 0+e 0+e],[0 1 1 1-e 1-e 0+e],c3);plot([0 1 1 0 0],[0 0 1 1 0]);disp('weights');
  "IW{2,1}(6,:)'" : Constant  Value=[0.8789095583685544443852677432005293667316436767578125;0.1033328624612124269077639837632887065410614013671875;0.21495730780066413245776857365854084491729736328125;0.258154889464636827511867522844113409519195556640625;-0.6675872790815227109106899661128409206867218017578125;-0.7209230739663452514065511422813870012760162353515625;-0.609485069906721577126518241129815578460693359375;-0.88092575992821853247960461885668337345123291015625;0.40496519285165444301810566685162484645843505859375;0.5625742905241113422931675813742913305759429931640625;0.0463479002260569483695462622563354671001434326171875;0.6352921530260806637357973158941604197025299072265625;0.53087459086909749572669170447625219821929931640625;0.7025753346407059840572628672816790640354156494140625;-0.3770567280982621838347768061794340610504150390625;-0.6860655094816063837015462922863662242889404296875;-0.72803056045027059184349127463065087795257568359375;0.3598736062536123103683394219842739403247833251953125;-0.9389672098291452773111132046324200928211212158203125;-0.43684369829937441664924335782416164875030517578125]
      mask Display: e = 0.06;c1 = [120 150 230]/255;c2 = ([120 150 230]+0)/383;c3 = ([120 150 230]+128)/383;patch([0 1 1 0],[0 0 1 1],c1);patch([0 1 1 1-e 1-e 0+e],[0 0 1 1-e 0+e 0+e],c2);patch([0 0 1 1-e 0+e 0+e],[0 1 1 1-e 1-e 0+e],c3);plot([0 1 1 0 0],[0 0 1 1 0]);disp('weights');
  "IW{2,1}(7,:)'" : Constant  Value=[0.342083827939231921444473982774070464074611663818359375;0.00120151092506673028321995122524867838365025818347930908203125;0.043697026340244506104060207007933058775961399078369140625;-0.90563919972410322767331081195152364671230316162109375;-0.319391809113331592850926199389505200088024139404296875;-0.23259452632812449568433521562837995588779449462890625;-0.150126226511819282904980354942381381988525390625;0.87592612371778122426491108853952027857303619384765625;-0.277046750542504660597131760368938557803630828857421875;-0.1816987017693799943973687049947329796850681304931640625;-0.62929130819107303995707525245961733162403106689453125;-0.1671130743117361927563280232789111323654651641845703125;-0.1846257842541703109162654072861187160015106201171875;0.50970962992658563894821099893306382000446319580078125;0.34035915582880249541375405897269956767559051513671875;-0.193717893315243638863165642760577611625194549560546875;-0.233682558501247694682234623542171902954578399658203125;0.87411360118726744161676833755336701869964599609375;0.267100451571945729511980971437878906726837158203125;-0.131499425922746271400143314167507924139499664306640625]
      mask Display: e = 0.06;c1 = [120 150 230]/255;c2 = ([120 150 230]+0)/383;c3 = ([120 150 230]+128)/383;patch([0 1 1 0],[0 0 1 1],c1);patch([0 1 1 1-e 1-e 0+e],[0 0 1 1-e 0+e 0+e],c2);patch([0 0 1 1-e 0+e 0+e],[0 1 1 1-e 1-e 0+e],c3);plot([0 1 1 0 0],[0 0 1 1 0]);disp('weights');
  "IW{2,1}(8,:)'" : Constant  Value=[-0.469976297641904405821833279333077371120452880859375;-0.345940942441360699266539313612156547605991363525390625;-0.54204101239868440753610911997384391725063323974609375;0.298804979050913299687408652971498668193817138671875;-0.80349891185214172839579305218649096786975860595703125;0.0862397587164498158340819600198301486670970916748046875;0.074152857735117816417869107681326568126678466796875;-0.60368017712577637379212092128000222146511077880859375;0.28771166324430286209690166288055479526519775390625;0.6793319094640664079776115613640286028385162353515625;-0.094607429192425485098283388651907444000244140625;0.6631891833519281131970046772039495408535003662109375;-0.562709031809010884472854741034097969532012939453125;0.048601955277117969700384492170996963977813720703125;0.054990383731804613753890720317940576933324337005615234375;-0.1480929533941710285471771157972398214042186737060546875;-0.07207754281066970636349111600793548859655857086181640625;0.27282035125016790289009804837405681610107421875;-0.2334247263419737816736443392073852010071277618408203125;-0.180121758537853449144705564322066493332386016845703125]
      mask Display: e = 0.06;c1 = [120 150 230]/255;c2 = ([120 150 230]+0)/383;c3 = ([120 150 230]+128)/383;patch([0 1 1 0],[0 0 1 1],c1);patch([0 1 1 1-e 1-e 0+e],[0 0 1 1-e 0+e 0+e],c2);patch([0 0 1 1-e 0+e 0+e],[0 1 1 1-e 1-e 0+e],c3);plot([0 1 1 0 0],[0 0 1 1 0]);disp('weights');
  "IW{2,1}(9,:)'" : Constant  Value=[0.556199631376198322385562278213910758495330810546875;-0.638202814113372429716264377930201590061187744140625;0.80842128477482499970818707879516296088695526123046875;0.1705050567257683502564447053373442031443119049072265625;0.896926001035158293461790890432894229888916015625;-0.861333575818907792864820294198580086231231689453125;-0.05476088910984468205445097055417136289179325103759765625;-0.897995772378146650538610629155300557613372802734375;-0.7421458016951871794475437127402983605861663818359375;0.367744587945827705599555201843031682074069976806640625;0.9086736653698832544279184730839915573596954345703125;-0.14915785778446688514264906189055182039737701416015625;-0.046113967678458940568919643965273280628025531768798828125;-0.7967495895263521088480729304137639701366424560546875;0.0294475795236336067295379592678727931343019008636474609375;0.89700051566761229704383140415302477777004241943359375;-0.468436386820892225468782044117688201367855072021484375;0.267801927749805546152828128469991497695446014404296875;0.572549028263678483341436731279827654361724853515625;0.69139723139074849012075674181687645614147186279296875]
      mask Display: e = 0.06;c1 = [120 150 230]/255;c2 = ([120 150 230]+0)/383;c3 = ([120 150 230]+128)/383;patch([0 1 1 0],[0 0 1 1],c1);patch([0 1 1 1-e 1-e 0+e],[0 0 1 1-e 0+e 0+e],c2);patch([0 0 1 1-e 0+e 0+e],[0 1 1 1-e 1-e 0+e],c3);plot([0 1 1 0 0],[0 0 1 1 0]);disp('weights');
  Mux : Mux  Inputs=20
      mask Display: e = 0.06;c1 = [120 150 230]/255;c2 = ([120 150 230]+0)/383;c3 = ([120 150 230]+128)/383;patch([0 1 1 0],[0 0 1 1],c1);patch([0 1 1 1-e 1-e 0+e],[0 0 1 1-e 0+e 0+e],c2);patch([0 0 1 1-e 0+e 0+e],[0 1 1 1-e 1-e 0+e],c3);plot([0 1 1 0 0],[0 0 1 1 0]);disp('Mux');
  dotprod{1..20} (20 alike) : neural/Weight Functions/dotprod
  "lz{2,1}" : Outport
      mask Display: e = 0.06;c1 = [120 230 180]/255;c2 = ([120 230 180]+0)/(256+128);c3 = ([120 230 180]+128)/(256+128);patch([0 1 1 0],[0 0 1 1],c1);patch([0 1 1 1-e 1-e 0+e],[0 0 1 1-e 0+e 0+e],c2);patch([0 0 1 1-e 0+e 0+e],[0 1 1 1-e 1-e 0+e],c3);plot([0 1 1 0 0],[0 0 1 1 0]);
  wires:
  Mux/1 -> "lz{2,1}"/1
  dotprod20/1 -> Mux/20
  "IW{2,1}(20,:)'"/1 -> dotprod20/1
  dotprod19/1 -> Mux/19
  "IW{2,1}(19,:)'"/1 -> dotprod19/1
  dotprod18/1 -> Mux/18
  "IW{2,1}(18,:)'"/1 -> dotprod18/1
  dotprod17/1 -> Mux/17
  "IW{2,1}(17,:)'"/1 -> dotprod17/1
  dotprod16/1 -> Mux/16
  "IW{2,1}(16,:)'"/1 -> dotprod16/1
  dotprod15/1 -> Mux/15
  "IW{2,1}(15,:)'"/1 -> dotprod15/1
  dotprod14/1 -> Mux/14
  "IW{2,1}(14,:)'"/1 -> dotprod14/1
  dotprod13/1 -> Mux/13
  "IW{2,1}(13,:)'"/1 -> dotprod13/1
  dotprod12/1 -> Mux/12
  "IW{2,1}(12,:)'"/1 -> dotprod12/1
  dotprod11/1 -> Mux/11
  "IW{2,1}(11,:)'"/1 -> dotprod11/1
  dotprod10/1 -> Mux/10
  "IW{2,1}(10,:)'"/1 -> dotprod10/1
  dotprod9/1 -> Mux/9
  "IW{2,1}(9,:)'"/1 -> dotprod9/1
  dotprod8/1 -> Mux/8
  "IW{2,1}(8,:)'"/1 -> dotprod8/1
  dotprod7/1 -> Mux/7
  "IW{2,1}(7,:)'"/1 -> dotprod7/1
  dotprod6/1 -> Mux/6
  "IW{2,1}(6,:)'"/1 -> dotprod6/1
  dotprod5/1 -> Mux/5
  "IW{2,1}(5,:)'"/1 -> dotprod5/1
  dotprod4/1 -> Mux/4
  "IW{2,1}(4,:)'"/1 -> dotprod4/1
  dotprod3/1 -> Mux/3
  "IW{2,1}(3,:)'"/1 -> dotprod3/1
  dotprod2/1 -> Mux/2
  "IW{2,1}(2,:)'"/1 -> dotprod2/1
  dotprod1/1 -> Mux/1
  "ad{2,1}"/1 -> dotprod20/2, dotprod19/2, dotprod18/2, dotprod17/2, dotprod16/2, dotprod15/2, dotprod14/2, dotprod13/2, dotprod12/2, dotprod11/2, dotprod10/2, dotprod9/2, dotprod8/2, dotprod7/2, dotprod6/2, dotprod5/2, dotprod4/2, dotprod3/2, dotprod2/2, dotprod1/2
  "IW{2,1}(1,:)'"/1 -> dotprod1/1

== system ClosedLoop/Controller 5x20/Layer 3/Delays 1 ==
  "p{3}" : Inport  PortDimensions=20
      mask Display: e = 0.06;c1 = [120 230 180]/255;c2 = ([120 230 180]+0)/(256+128);c3 = ([120 230 180]+128)/(256+128);patch([0 1 1 0],[0 0 1 1],c1);patch([0 1 1 1-e 1-e 0+e],[0 0 1 1-e 0+e 0+e],c2);patch([0 0 1 1-e 0+e 0+e],[0 1 1 1-e 1-e 0+e],c3);plot([0 1 1 0 0],[0 0 1 1 0]);
  mux : Mux  Inputs=1
      mask Display: e = 0.06;c1 = [120 150 230]/255;c2 = ([120 150 230]+0)/383;c3 = ([120 150 230]+128)/383;patch([0 1 1 0],[0 0 1 1],c1);patch([0 1 1 1-e 1-e 0+e],[0 0 1 1-e 0+e 0+e],c2);patch([0 0 1 1-e 0+e 0+e],[0 1 1 1-e 1-e 0+e],c3);plot([0 1 1 0 0],[0 0 1 1 0]);disp('Mux')
  "pd{3,2}" : Outport
      mask Display: e = 0.06;c1 = [120 230 180]/255;c2 = ([120 230 180]+0)/(256+128);c3 = ([120 230 180]+128)/(256+128);patch([0 1 1 0],[0 0 1 1],c1);patch([0 1 1 1-e 1-e 0+e],[0 0 1 1-e 0+e 0+e],c2);patch([0 0 1 1-e 0+e 0+e],[0 1 1 1-e 1-e 0+e],c3);plot([0 1 1 0 0],[0 0 1 1 0]);
  wires:
  mux/1 -> "pd{3,2}"/1
  "p{3}"/1 -> mux/1
